simulink model "Surface_model_Simulink"  (R2022a)
settings: Solver=VariableStepAuto  StartTime=0.0  StopTime=10.0  RelTol=1e-3
values from neighbouring files (symbols this model uses):
  d = 1    [main_surface_bot_model.m]
  Izz = 2348.97    [main_surface_bot_model.m]
  m = 1462    [main_surface_bot_model.m]
settings Model: Creator=G_Sushmanth_Sai  LastModifiedBy=G_Sushmanth_Sai

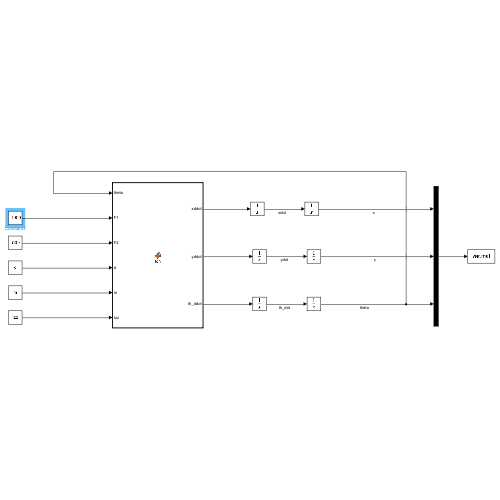
[thumbnail: Simulink's stored preview of the top-level diagram]
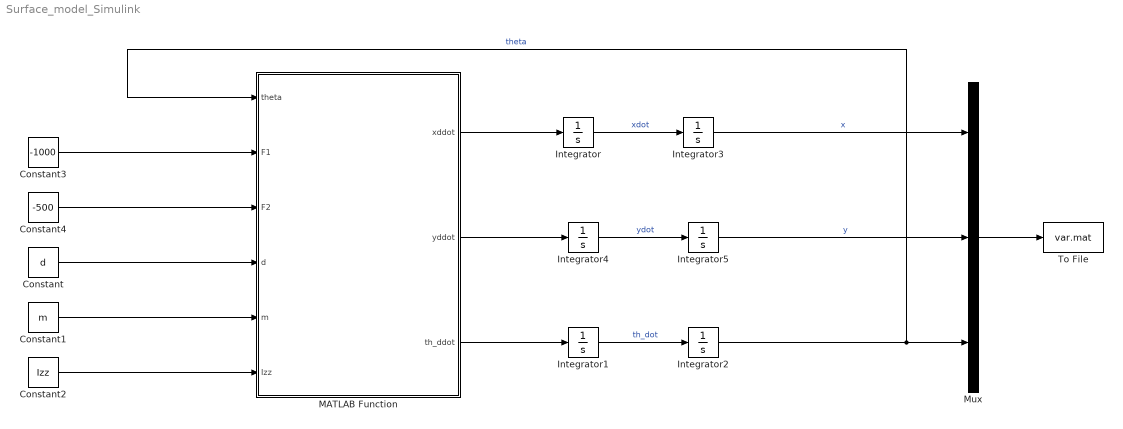
== system Surface_model_Simulink ==
  Constant : Constant  Value=d
  Constant1 : Constant  Value=m
  Constant2 : Constant  Value=Izz
  Constant3 : Constant  Value=-1000
  Constant4 : Constant  Value=-500
  Integrator{,1..5} (6 alike) : Integrator
  MATLAB Function : MATLAB Function  TreatAsAtomicUnit=on
  Mux : Mux  Inputs=3
  To File : ToFile  Filename=var.mat  MatrixName=tot
  wires:
  Integrator1/1 -> Integrator2/1  "th_dot"
  Integrator/1 -> Integrator3/1  "xdot"
  Integrator3/1 -> Mux/1  "x"
  Constant4/1 -> MATLAB Function/3(F2)
  Constant3/1 -> MATLAB Function/2(F1)
  Constant/1 -> MATLAB Function/4(d)
  Constant1/1 -> MATLAB Function/5(m)
  Constant2/1 -> MATLAB Function/6(Izz)
  Integrator5/1 -> Mux/2  "y"
  Integrator4/1 -> Integrator5/1  "ydot"
  MATLAB Function/1(xddot) -> Integrator/1
  MATLAB Function/2(yddot) -> Integrator4/1
  MATLAB Function/3(th_ddot) -> Integrator1/1
  Integrator2/1 -> Mux/3, MATLAB Function/1(theta)  "theta"
  Mux/1 -> To File/1

== matlab function Surface_model_Simulink/MATLAB Function ==
  data: theta input; xddot output; F1 input; F2 input; d input; m input; yddot output; th_ddot output; Izz input
function [xddot,yddot,th_ddot] = fcn(theta, F1, F2, d, m, Izz)

xddot = -(F1+F2)*cos(theta)/m;
yddot = -(F1+F2)*sin(theta)/m;
th_ddot = -(F2 - F1)*(d/(2*Izz));

end
